simulink model "sampleModel1650"  (R2023a)
settings: Solver=VariableStepAuto  StartTime=0.0  StopTime=10.0  RelTol=1e-3
libraries: hdlsllib x5
settings Model: Creator=user1  LastModifiedBy=user1

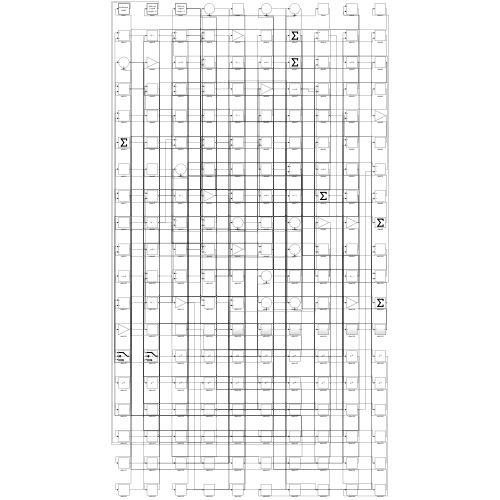
[thumbnail: Simulink's stored preview of the top-level diagram]
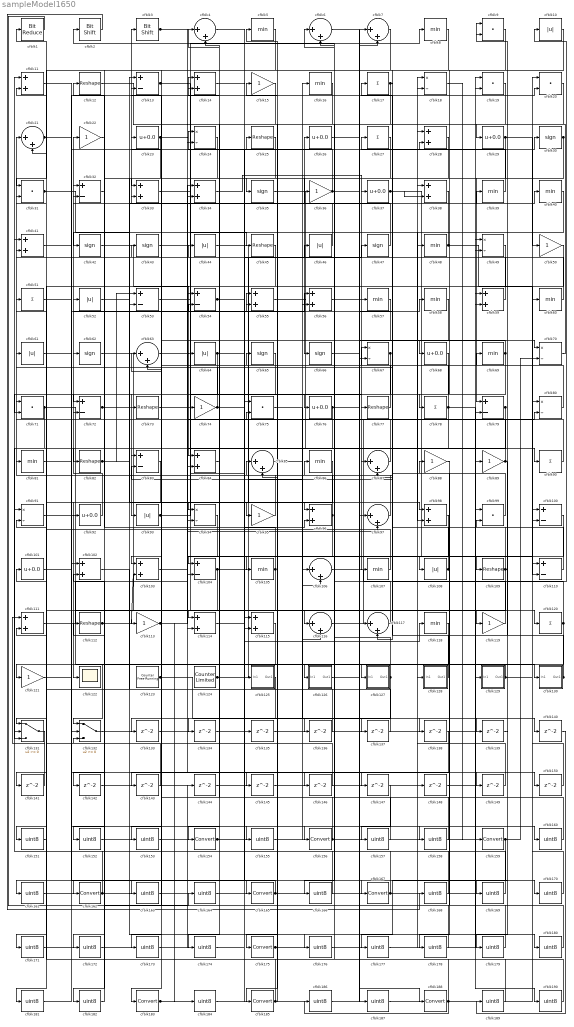
== system sampleModel1650 ==
  cfblk1 : hdlsllib/Logic and Bit Operations/Bit Reduce  mode=AND
  cfblk{10,44,46,52,61,64,93,108} (8 alike) : Abs  SaturateOnIntegerOverflow=off
  cfblk{13,32,53..54,72,79,83,100,104,110} (10 alike) : Sum  Inputs=+-
  cfblk{23,26,29,37,68,76,92,101} (8 alike) : Bias  Bias=0.0  SaturateOnIntegerOverflow=off
  cfblk{11,14,28,33..34,38,41,55..56,59,84,96,98,102..103,111,114..115} (18 alike) : Sum
  cfblk{5,8,16,39..40,48,57..58,60,69,81,86,105,107,118} (15 alike) : MinMax
  cfblk{4,6..7,21,63,85,87,97,106,116..117} (11 alike) : Sum  Inputs=|++
  cfblk{12,25,45,73,77,82,109,112} (8 alike) : Reshape
  cfblk{15,22,36,50,74,88..89,95,113,119,121} (11 alike) : Gain
  cfblk{17,27,51,78,90,120} (6 alike) : Sum  Inputs=+
  cfblk122 : Scope
  cfblk123 : hdlsllib/Sources/Counter Free-Running  NumBits=16  tsamp=-1
  cfblk124 : hdlsllib/Sources/Counter Limited  uplimit=7  tsamp=-1
  cfblk125 : Subsystem
      settings: LibrarySourceBlock=|
      | hdlsllib/Ports &
      | Subsystems/Subsystem
  cfblk126 : Subsystem
      settings: LibrarySourceBlock=|
      | hdlsllib/Ports &
      | Subsystems/Subsystem
  cfblk127 : Subsystem
      settings: LibrarySourceBlock=|
      | hdlsllib/Ports &
      | Subsystems/Subsystem
  cfblk128 : Subsystem
      settings: LibrarySourceBlock=|
      | hdlsllib/Ports &
      | Subsystems/Subsystem
  cfblk129 : Subsystem
      settings: LibrarySourceBlock=|
      | hdlsllib/Ports &
      | Subsystems/Subsystem
  cfblk130 : Subsystem
      settings: LibrarySourceBlock=|
      | hdlsllib/Ports &
      | Subsystems/Subsystem
  cfblk131 : Switch  SaturateOnIntegerOverflow=off  InputSameDT=off
  cfblk132 : Switch  SaturateOnIntegerOverflow=off  InputSameDT=off
  cfblk{133..150} (18 alike) : Delay  SampleTime=1
  cfblk{151..153,155,157..158,160..161,163..164,166,168..174,176..182,184,186..187,189..190} (30 alike) : DataTypeConversion  OutDataTypeStr=uint8  SaturateOnIntegerOverflow=off  RndMeth=Floor
  cfblk{154,156,159,162,165,167,175,183,185,188} (10 alike) : DataTypeConversion  SaturateOnIntegerOverflow=off  RndMeth=Floor
  cfblk{18,24,49,67,70,80,91,94} (8 alike) : Product  Inputs=*/  RndMeth=Zero  SaturateOnIntegerOverflow=on
  cfblk{9,19..20,31,71,75,99} (7 alike) : DotProduct  OutDataTypeStr=Inherit: Inherit via internal rule
  cfblk2 : hdlsllib/Logic and Bit Operations/Bit Shift  mode=Shift Left Logical  N=0
  cfblk3 : hdlsllib/Logic and Bit Operations/Bit Shift  mode=Shift Left Logical  N=0
  cfblk{30,35,42..43,47,62,65..66} (8 alike) : Signum
  wires:
  cfblk30/1 -> cfblk79/1, cfblk107/1
  cfblk120/1 -> cfblk127/1(In1), cfblk99/2
  cfblk70/1 -> cfblk29/1
  cfblk6/1 -> cfblk188/1
  cfblk124/1 -> cfblk35/1, cfblk118/1
  cfblk82/1 -> cfblk53/1, cfblk94/1
  cfblk37/1 -> cfblk109/1, cfblk38/2
  cfblk95/1 -> cfblk21/1
  cfblk92/1 -> cfblk22/1
  cfblk34/1 -> cfblk108/1
  cfblk46/1 -> cfblk26/1
  cfblk60/1 -> cfblk5/1
  cfblk5/1 -> cfblk31/1
  cfblk13/1 -> cfblk120/1, cfblk150/1
  cfblk74/1 -> cfblk61/1, cfblk160/1
  cfblk24/1 -> cfblk53/2
  cfblk83/1 -> cfblk122/1
  cfblk15/1 -> cfblk154/1
  cfblk106/1 -> cfblk10/1
  cfblk71/1 -> cfblk126/1(In1), cfblk131/2
  cfblk33/1 -> cfblk77/1
  cfblk62/1 -> cfblk119/1
  cfblk99/1 -> cfblk62/1
  cfblk129/1(Out1) -> cfblk60/1, cfblk121/1
  cfblk53/1 -> cfblk8/1
  cfblk44/1 -> cfblk98/1
  cfblk47/1 -> cfblk3/1
  cfblk76/1 -> cfblk149/1, cfblk152/1
  cfblk68/1 -> cfblk93/1
  cfblk130/1(Out1) -> cfblk52/1, cfblk9/2
  cfblk93/1 -> cfblk39/1, cfblk28/2
  cfblk57/1 -> cfblk183/1
  cfblk89/1 -> cfblk65/1, cfblk69/1, cfblk179/1
  cfblk118/1 -> cfblk132/1
  cfblk50/1 -> cfblk84/1
  cfblk19/1 -> cfblk175/1
  cfblk39/1 -> cfblk27/1
  cfblk109/1 -> cfblk9/1, cfblk72/2, cfblk171/1
  cfblk96/1 -> cfblk81/1, cfblk174/1
  cfblk28/1 -> cfblk33/1
  cfblk12/1 -> cfblk84/2
  cfblk77/1 -> cfblk32/1
  cfblk48/1 -> cfblk42/1, cfblk110/1
  cfblk31/1 -> cfblk73/1, cfblk30/1
  cfblk91/1 -> cfblk116/1
  cfblk42/1 -> cfblk74/1
  cfblk119/1 -> cfblk67/1
  cfblk97/1 -> cfblk86/1
  cfblk113/1 -> cfblk80/2, cfblk184/1
  cfblk84/1 -> cfblk24/1
  cfblk7/1 -> cfblk162/1
  cfblk87/1 -> cfblk12/1
  cfblk73/1 -> cfblk34/1
  cfblk58/1 -> cfblk103/1
  cfblk117/1 -> cfblk71/1
  cfblk123/1 -> cfblk33/2, cfblk187/1
  cfblk116/1 -> cfblk59/1
  cfblk65/1 -> cfblk71/2
  cfblk128/1(Out1) -> cfblk85/1
  cfblk55/1 -> cfblk90/1
  cfblk121/1 -> cfblk55/1
  cfblk3/1 -> cfblk87/1, cfblk130/1(In1), cfblk97/2
  cfblk22/1 -> cfblk82/1
  cfblk17/1 -> cfblk117/2, cfblk146/1
  cfblk132/1 -> cfblk79/2
  cfblk90/1 -> cfblk17/1
  cfblk79/1 -> cfblk85/2, cfblk131/3
  cfblk35/1 -> cfblk129/1(In1)
  cfblk26/1 -> cfblk70/1
  cfblk27/1 -> cfblk66/1
  cfblk18/1 -> cfblk159/1
  cfblk107/1 -> cfblk51/1
  cfblk4/1 -> cfblk156/1
  cfblk103/1 -> cfblk54/1
  cfblk78/1 -> cfblk44/1, cfblk133/1, cfblk190/1
  cfblk127/1(Out1) -> cfblk2/1, cfblk153/1
  cfblk105/1 -> cfblk32/2, cfblk143/1, cfblk182/1
  cfblk20/1 -> cfblk37/1
  cfblk111/1 -> cfblk34/2
  cfblk104/1 -> cfblk36/1, cfblk114/1, cfblk96/2
  cfblk21/1 -> cfblk145/1, cfblk158/1
  cfblk110/1 -> cfblk43/1
  cfblk63/1 -> cfblk55/2
  cfblk40/1 -> cfblk98/2
  cfblk94/1 -> cfblk104/1
  cfblk85/1 -> cfblk16/1
  cfblk67/1 -> cfblk114/2, cfblk166/1
  cfblk59/1 -> cfblk11/2
  cfblk38/1 -> cfblk76/1
  cfblk126/1(Out1) -> cfblk97/1
  cfblk9/1 -> cfblk87/2
  cfblk43/1 -> cfblk45/1
  cfblk81/1 -> cfblk14/1
  cfblk98/1 -> cfblk104/2
  cfblk112/1 -> cfblk103/2, cfblk20/2
  cfblk72/1 -> cfblk40/1, cfblk95/1
  cfblk16/1 -> cfblk24/2
  cfblk51/1 -> cfblk54/2
  cfblk54/1 -> cfblk47/1, cfblk136/1
  cfblk23/1 -> cfblk92/1, cfblk110/2
  cfblk64/1 -> cfblk131/1, cfblk56/1, cfblk72/1
  cfblk10/1 -> cfblk78/1
  cfblk108/1 -> cfblk105/1, cfblk83/2
  cfblk66/1 -> cfblk58/1
  cfblk131/1 -> cfblk111/1
  cfblk41/1 -> cfblk167/1
  cfblk80/1 -> cfblk13/2
  cfblk25/1 -> cfblk113/1
  cfblk29/1 -> cfblk50/1, cfblk68/1
  cfblk56/1 -> cfblk117/1
  cfblk69/1 -> cfblk64/1, cfblk94/2, cfblk173/1
  cfblk100/1 -> cfblk185/1
  cfblk52/1 -> cfblk96/1
  cfblk8/1 -> cfblk83/1
  cfblk101/1 -> cfblk165/1
  cfblk36/1 -> cfblk14/2, cfblk139/1
  cfblk133/1 -> cfblk116/2
  cfblk125/1(Out1) -> cfblk134/1
  cfblk134/1 -> cfblk59/2
  cfblk135/1 -> cfblk106/2
  cfblk136/1 -> cfblk13/1
  cfblk14/1 -> cfblk137/1
  cfblk137/1 -> cfblk1/1
  cfblk75/1 -> cfblk138/1
  cfblk114/1 -> cfblk140/1
  cfblk45/1 -> cfblk141/1
  cfblk141/1 -> cfblk11/1
  cfblk32/1 -> cfblk142/1
  cfblk142/1 -> cfblk28/1
  cfblk143/1 -> cfblk91/2
  cfblk145/1 -> cfblk67/2
  cfblk146/1 -> cfblk63/1
  cfblk61/1 -> cfblk147/1
  cfblk148/1 -> cfblk99/1
  cfblk149/1 -> cfblk38/1
  cfblk150/1 -> cfblk80/1
  cfblk49/1 -> cfblk151/1
  cfblk151/1 -> cfblk31/2
  cfblk152/1 -> cfblk49/1
  cfblk153/1 -> cfblk49/2
  cfblk154/1 -> cfblk56/2, cfblk128/1(In1), cfblk106/1
  cfblk11/1 -> cfblk155/1
  cfblk155/1 -> cfblk15/1
  cfblk156/1 -> cfblk48/1, cfblk63/2
  cfblk147/1 -> cfblk157/1
  cfblk157/1 -> cfblk4/1
  cfblk158/1 -> cfblk4/2
  cfblk159/1 -> cfblk70/2, cfblk177/1
  cfblk160/1 -> cfblk18/1
  cfblk161/1 -> cfblk18/2
  cfblk162/1 -> cfblk91/1, cfblk176/1
  cfblk138/1 -> cfblk163/1
  cfblk163/1 -> cfblk7/1
  cfblk1/1 -> cfblk164/1
  cfblk164/1 -> cfblk7/2
  cfblk165/1 -> cfblk161/1, cfblk89/1
  cfblk166/1 -> cfblk101/1
  cfblk167/1 -> cfblk132/3, cfblk132/2, cfblk46/1
  cfblk2/1 -> cfblk168/1
  cfblk168/1 -> cfblk41/1
  cfblk139/1 -> cfblk169/1
  cfblk169/1 -> cfblk41/2
  cfblk144/1 -> cfblk170/1
  cfblk170/1 -> cfblk20/1
  cfblk171/1 -> cfblk144/1
  cfblk115/1 -> cfblk172/1
  cfblk172/1 -> cfblk75/1
  cfblk173/1 -> cfblk115/1
  cfblk174/1 -> cfblk115/2
  cfblk175/1 -> cfblk148/1, cfblk75/2
  cfblk176/1 -> cfblk19/1
  cfblk177/1 -> cfblk19/2
  cfblk88/1 -> cfblk178/1
  cfblk178/1 -> cfblk112/1
  cfblk179/1 -> cfblk88/1
  cfblk102/1 -> cfblk180/1
  cfblk180/1 -> cfblk23/1
  cfblk86/1 -> cfblk181/1
  cfblk181/1 -> cfblk102/1
  cfblk182/1 -> cfblk102/2
  cfblk183/1 -> cfblk135/1, cfblk125/1(In1)
  cfblk184/1 -> cfblk57/1
  cfblk185/1 -> cfblk111/2, cfblk25/1
  cfblk186/1 -> cfblk100/1
  cfblk187/1 -> cfblk100/2
  cfblk188/1 -> cfblk186/1, cfblk21/2
  cfblk140/1 -> cfblk189/1
  cfblk189/1 -> cfblk6/1
  cfblk190/1 -> cfblk6/2

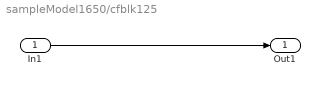
== system sampleModel1650/cfblk125 ==
  In1 : Inport
  Out1 : Outport
  wires:
  In1/1 -> Out1/1

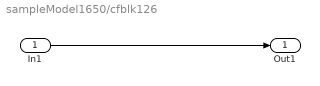
== system sampleModel1650/cfblk126 ==
  In1 : Inport
  Out1 : Outport
  wires:
  In1/1 -> Out1/1

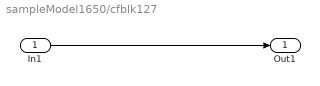
== system sampleModel1650/cfblk127 ==
  In1 : Inport
  Out1 : Outport
  wires:
  In1/1 -> Out1/1

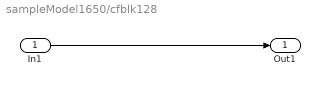
== system sampleModel1650/cfblk128 ==
  In1 : Inport
  Out1 : Outport
  wires:
  In1/1 -> Out1/1

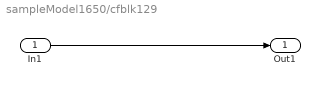
== system sampleModel1650/cfblk129 ==
  In1 : Inport
  Out1 : Outport
  wires:
  In1/1 -> Out1/1

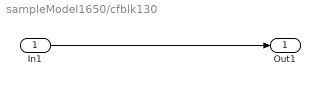
== system sampleModel1650/cfblk130 ==
  In1 : Inport
  Out1 : Outport
  wires:
  In1/1 -> Out1/1
